simulink model "nonlin_model_d_1"  (Simulink 6.4)
settings: Solver=ode45  StartTime=0.0  StopTime=0.01  FixedStep=0.0001  RelTol=1e-3
libraries: simulink x1
settings Model: Creator=dan  LastModifiedBy=dan  BufferReuse=off
settings DataIOCC: SignalLoggingName=sigsOut
settings OptimizationCC: InlineInvariantSignals=on  OptimizeBlockIOStorage=off  BufferReuse=off  ExpressionFolding=off  LocalBlockOutputs=off  InitFltsAndDblsToZero=off
settings DebuggingCC: SolverPrmCheckMsg=none  StrictBusMsg=None
settings HardwareCC: TargetHWDeviceType=32-bit Generic  TargetUnknown=on  ProdEqTarget=off

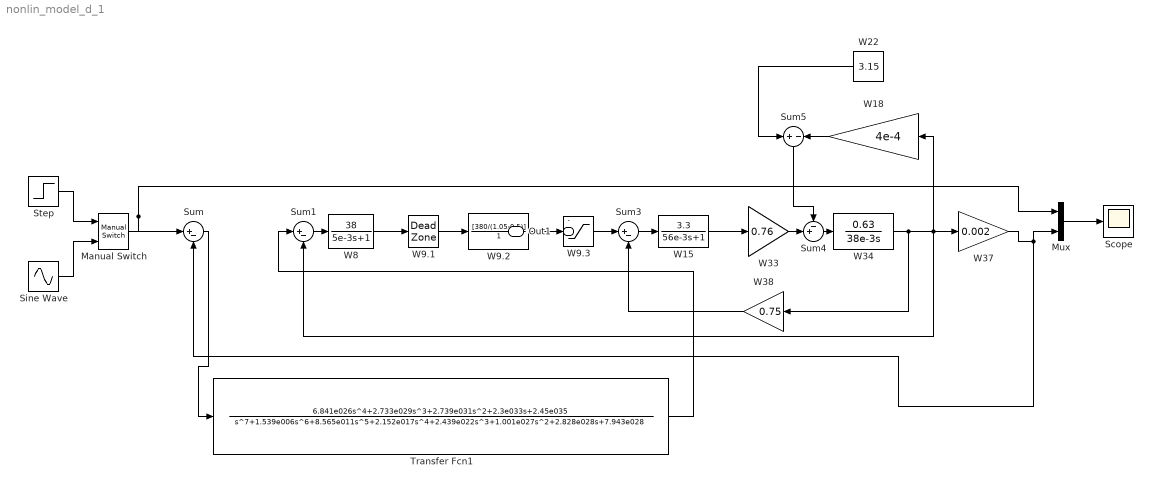
== system nonlin_model_d_1 ==
  Manual Switch : simulink/Signal Routing/Manual Switch  SystemSampleTime=-1  sw=1  action=0
  Mux : Mux  Inputs=2
  Scope : Scope
      settings: TimeRange=0.01  YMin=2.77556e-017  YMax=1
  Sine Wave : Sin  Amplitude=1  Bias=0  Frequency=1200  Phase=0  Samples=10  SampleTime=0  Offset=0
  Step : Step  Time=0  SampleTime=0
  Sum : Sum  Inputs=|+-  OutDataType=sfix(16)  OutScaling=2^0  SaturateOnIntegerOverflow=on
  Sum1 : Sum  Inputs=|+-  OutDataType=sfix(16)  OutScaling=2^0  SaturateOnIntegerOverflow=on
  Sum3 : Sum  Inputs=|+-  OutDataType=sfix(16)  OutScaling=2^0  SaturateOnIntegerOverflow=on
  Sum4 : Sum  Inputs=-+|  OutDataType=sfix(16)  OutScaling=2^0  SaturateOnIntegerOverflow=on
  Sum5 : Sum  Orientation=down  Inputs=+|-  OutDataType=sfix(16)  OutScaling=2^0  SaturateOnIntegerOverflow=on
  Transfer Fcn1 : TransferFcn  Numerator=[6.841e026 2.733e029 2.739e031 2.3e033 2.45e035]  Denominator=[1 1.539e006 8.565e011 2.152e017 2.439e022 1.001e027 2.828e028 7.943e028]
  W15 : TransferFcn  Numerator=[3.3]  Denominator=[56e-3 1]
  W18 : Gain  Orientation=left  Gain=4e-4  ParameterDataType=sfix(16)  ParameterScaling=2^0  OutDataType=sfix(16)  OutScaling=2^0  SaturateOnIntegerOverflow=on
  W22 : Constant  Orientation=left  Value=3.15  OutDataType=sfix(16)  OutScaling=2^0
  W33 : Gain  Gain=0.76  ParameterDataType=sfix(16)  ParameterScaling=2^0  OutDataType=sfix(16)  OutScaling=2^0  SaturateOnIntegerOverflow=on
  W34 : TransferFcn  Numerator=[0.63]  Denominator=[38e-3 0]
  W37 : Gain  Gain=0.002  ParameterDataType=sfix(16)  ParameterScaling=2^0  OutDataType=sfix(16)  OutScaling=2^0  SaturateOnIntegerOverflow=on
  W38 : Gain  Orientation=left  Gain=0.75  ParameterDataType=sfix(16)  ParameterScaling=2^0  OutDataType=sfix(16)  OutScaling=2^0  SaturateOnIntegerOverflow=on
  W8 : TransferFcn  Numerator=[38]  Denominator=[5e-3 1]
  W9.1 : DeadZone  LowerValue=-0.6  UpperValue=0.6  SaturateOnIntegerOverflow=on
  W9.2 : TransferFcn  Numerator=[380/(1.05-0.5)]  Denominator=[1]
  W9.3 : Saturate  UpperLimit=380  LowerLimit=-380
  . : Outport
  Out1 : Outport  Port=2
  wires:
  Step/1 -> Manual Switch/1
  Sine Wave/1 -> Manual Switch/2
  Mux/1 -> Scope/1
  Manual Switch/1 -> Mux/1, Sum/1
  Sum3/1 -> W15/1
  W15/1 -> W33/1
  W34/1 -> W38/1, W37/1, Sum1/2, W18/1
  W37/1 -> Sum/2, Mux/2
  W38/1 -> Sum3/2
  Sum1/1 -> W9.2/1, W8/1
  Sum/1 -> Transfer Fcn1/1
  Transfer Fcn1/1 -> Sum1/1
  Sum4/1 -> W34/1
  W33/1 -> Sum4/2
  W22/1 -> Sum5/1
  W8/1 -> W9.1/1
  W18/1 -> Sum5/2
  Sum5/1 -> Sum4/1
  W9.1/1 -> Sum3/1
  W9.2/1 -> W9.3/1
  W9.3/1 -> ./1
